simulink model "regulator_sistem_cu_timp_mort_cu_integrator"  (R2023b)
settings: Solver=VariableStepAuto  StartTime=0.0  StopTime=100  MaxStep=1e-3  RelTol=1e-3
values from neighbouring files (symbols this model uses):
  den = [T 1]    [sns_proiect_Ceoca_Ovidiu.m]
  num = [1]    [sns_proiect_Ceoca_Ovidiu.m]
  taum = 1    [sns_proiect_Ceoca_Ovidiu.m]
undefined symbols (not defined in the file or in its folder): Kp_ZN, Ti_ZN
settings Model: Creator=ovidiuceoca  LastModifiedBy=ovidiuceoca

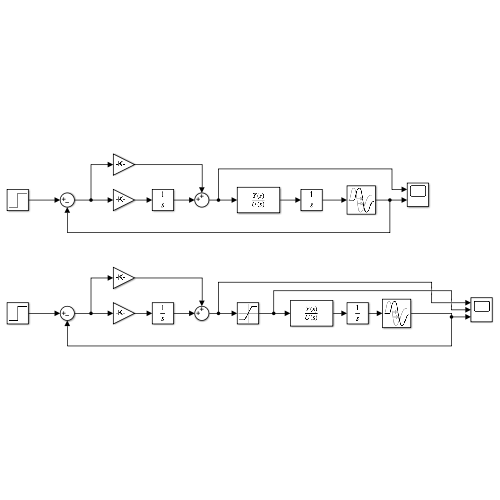
[thumbnail: Simulink's stored preview of the top-level diagram]
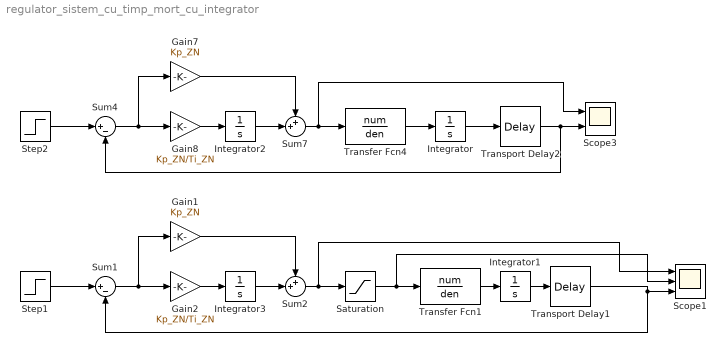
== system regulator_sistem_cu_timp_mort_cu_integrator ==
  Gain1 : Gain  Gain=Kp_ZN
  Gain2 : Gain  Gain=Kp_ZN/Ti_ZN
  Gain7 : Gain  Gain=Kp_ZN
  Gain8 : Gain  Gain=Kp_ZN/Ti_ZN
  Integrator{,1..3} (4 alike) : Integrator
  Saturation : Saturate  UpperLimit=1.2  LowerLimit=-1
  Scope1 : Scope  NumInputPorts=3
  Scope3 : Scope  NumInputPorts=2
  Step1 : Step  Time=0  SampleTime=0
  Step2 : Step  Time=0  SampleTime=0
  Sum1 : Sum  Inputs=|+-
  Sum2 : Sum  Inputs=++|
  Sum4 : Sum  Inputs=|+-
  Sum7 : Sum  Inputs=++|
  Transfer Fcn1 : TransferFcn  Numerator=num  Denominator=den
  Transfer Fcn4 : TransferFcn  Numerator=num  Denominator=den
  Transport Delay1 : TransportDelay  DelayTime=taum
  Transport Delay2 : TransportDelay  DelayTime=taum
  wires:
  Transport Delay2/1 -> Sum4/2, Scope3/2
  Step2/1 -> Sum4/1
  Gain8/1 -> Integrator2/1
  Sum4/1 -> Gain7/1, Gain8/1
  Sum7/1 -> Scope3/1, Transfer Fcn4/1
  Gain7/1 -> Sum7/1
  Integrator2/1 -> Sum7/2
  Transfer Fcn4/1 -> Integrator/1
  Integrator/1 -> Transport Delay2/1
  Sum2/1 -> Scope1/1, Saturation/1
  Sum1/1 -> Gain1/1, Gain2/1
  Transfer Fcn1/1 -> Integrator1/1
  Integrator1/1 -> Transport Delay1/1
  Gain2/1 -> Integrator3/1
  Integrator3/1 -> Sum2/2
  Transport Delay1/1 -> Sum1/2, Scope1/3
  Gain1/1 -> Sum2/1
  Step1/1 -> Sum1/1
  Saturation/1 -> Scope1/2, Transfer Fcn1/1
